simulink model "TestFlightMode"  (R2016a)
settings: Solver=FixedStepAuto  StartTime=0.0  StopTime=inf  RelTol=1e-3
libraries: SimuCopterToolbox x3
settings Model: SimulationMode=external  Creator=IceDragon  LastModifiedBy=hanan
settings SolverCC: PositivePriorityOrder=on
settings OptimizationCC: OptimizeModelRefInitCode=on  LifeSpan=1  MaxStackSize=64
settings HardwareCC: ProdBitPerPointer=32  ProdLargestAtomicInteger=Long  ProdLargestAtomicFloat=Double  ProdWordSize=32  ProdHWDeviceType=ARM Compatible->ARM Cortex
settings RTWCC: SystemTargetFile=ert.tlc  HardwareBoard=Raspberry Pi  TemplateMakefile=ert_default_tmf  CustomInclude=bridge simucopter  CustomSource=simucopter-agent.cpp BridgeClient.cpp ZmqBridgeMessageSerializer.cpp AbstractBridgeCommandHandler.cpp BridgeMessage.cpp  CustomDefine=SIMULINK_AGENT  CustomInitializer=simucopter_init();  CustomTerminator=simucopter_stop();  Toolchain=GNU GCC Raspberry Pi  BuildConfiguration=Specify  TargetLang=C++
settings CodeAppCC: ForceParamTrailComments=on  OperatorAnnotations=on  SimulinkDataObjDesc=on  SFDataObjDesc=on  MATLABFcnDesc=on  MangleLength=10  InsertBlockDesc=on  MATLABSourceComments=on
settings ERTTargetCC: SupportVariableSizeSignals=on  ExtModeMexArgs='10.66.66.254' 0 17725  RootIOFormat=Structure reference  IndentSize=4

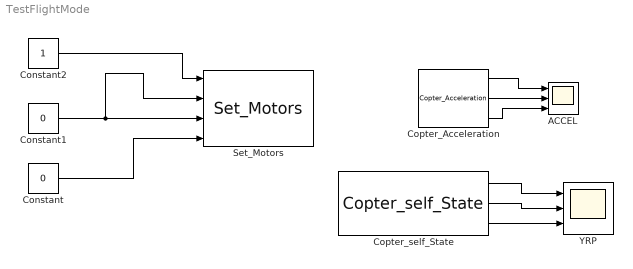
== system TestFlightMode ==
  ACCEL : Scope  NumInputPorts=3
  Constant : Constant  Value=0
  Constant1 : Constant  Value=0
  Constant2 : Constant
  Copter_Acceleration : SimuCopterToolbox/Copter_Acceleration  SimulateUsing=Code generation
  Copter_self_State : SimuCopterToolbox/Copter_self_State  SimulateUsing=Code generation
  Set_Motors : SimuCopterToolbox/Set_Motors  SimulateUsing=Code generation
  YRP : Scope  NumInputPorts=3
  wires:
  Copter_Acceleration/1 -> ACCEL/1
  Copter_Acceleration/2 -> ACCEL/2
  Copter_Acceleration/3 -> ACCEL/3
  Constant/1 -> Set_Motors/4
  Constant1/1 -> Set_Motors/2, Set_Motors/3
  Copter_self_State/1 -> YRP/1
  Copter_self_State/2 -> YRP/2
  Copter_self_State/3 -> YRP/3
  Constant2/1 -> Set_Motors/1
